simulink model "dynamics"  (R2017b)
settings: Solver=VariableStepAuto  StartTime=0.0  StopTime=10.0  RelTol=1e-3
libraries: shared6dof x1
settings Model: Creator=DanAdmin  LastModifiedBy=DanAdmin

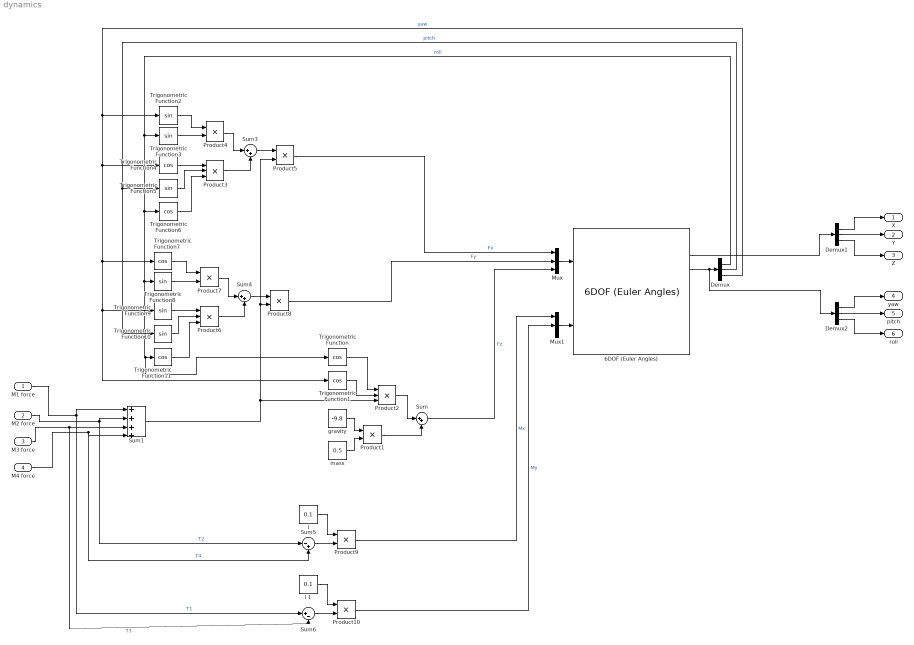
== system dynamics ==
  M1 force : Inport
  M2 force : Inport  Port=2
  M3 force : Inport  Port=3
  M4 force : Inport  Port=4
  6DOF (Euler Angles) : shared6dof/6DOF (Euler Angles)  units=Metric (MKS)  mtype=Fixed  rep=Euler Angles  xme_0=[0 0 0]  Vm_0=[0 0 0]  eul_0=[0 0 0]  pm_0=[0 0 0]  mass_0=1.0  mass_e=0.5  mass_f=2.0  inertia=eye(3)  inertia_e=eye(3)  inertia_f=2*eye(3)  k_quat=1.0  vre_flag=on  abi_flag=off
      settings: SourceProductBaseCode=AE
  Demux : Demux  Outputs=3
  Demux1 : Demux  Outputs=3
  Demux2 : Demux  Outputs=3
  Mux : Mux  Inputs=3
  Mux1 : Mux  Inputs=3
  Product{1,4..5,7..10} (7 alike) : Product
  Product2 : Product  Inputs=3
  Product3 : Product  Inputs=3
  Product6 : Product  Inputs=3
  Sum : Sum  Inputs=|++
  Sum1 : Sum  Inputs=|++++
  Sum3 : Sum  Inputs=|++
  Sum4 : Sum  Inputs=|++
  Sum5 : Sum  Inputs=|-+
  Sum6 : Sum  Inputs=|+-
  Trigonometric Function{,1,4,6..7,11} (6 alike) : Trigonometry  Operator=cos
  Trigonometric Function{2..3,5,8..10} (6 alike) : Trigonometry
  gravity : Constant  Value=-9.8
  "l " : Constant  Value=0.1
  l 1 : Constant  Value=0.1
  mass : Constant  Value=0.5
  X : Outport
  Y : Outport  Port=2
  Z : Outport  Port=3
  yaw : Outport  Port=4
  pitch : Outport  Port=5
  roll : Outport  Port=6
  wires:
  Mux/1 -> 6DOF (Euler Angles)/1
  Sum/1 -> Mux/3  "Fz"
  mass/1 -> Product1/2
  gravity/1 -> Product1/1
  Trigonometric Function/1 -> Product2/1
  Trigonometric Function1/1 -> Product2/2
  Product2/1 -> Sum/1
  6DOF (Euler Angles)/2 -> Demux1/1
  M1 force/1 -> Sum6/1, Sum1/1  "T1"
  M2 force/1 -> Sum5/1, Sum1/2  "T2"
  M4 force/1 -> Sum5/2, Sum1/4  "T4"
  Product1/1 -> Sum/2
  Product3/1 -> Sum3/2
  Product5/1 -> Mux/1  "Fx"
  Demux/1 -> Trigonometric Function/1, Trigonometric Function11/1, Trigonometric Function8/1, Trigonometric Function6/1, Trigonometric Function3/1  "roll"
  Trigonometric Function2/1 -> Product4/1
  Trigonometric Function3/1 -> Product4/2
  Product4/1 -> Sum3/1
  Trigonometric Function4/1 -> Product3/1
  Trigonometric Function5/1 -> Product3/2
  Trigonometric Function6/1 -> Product3/3
  Demux/2 -> Trigonometric Function10/1, Trigonometric Function5/1  "pitch"
  Sum3/1 -> Product5/1
  Product7/1 -> Sum4/1
  Product8/1 -> Mux/2  "Fy"
  Product6/1 -> Sum4/2
  Trigonometric Function10/1 -> Product6/2
  Sum1/1 -> Product8/2, Product5/2, Product2/3
  Trigonometric Function7/1 -> Product7/1
  Sum4/1 -> Product8/1
  Trigonometric Function8/1 -> Product7/2
  Trigonometric Function9/1 -> Product6/1
  Demux/3 -> Trigonometric Function1/1, Trigonometric Function9/1, Trigonometric Function7/1, Trigonometric Function4/1, Trigonometric Function2/1  "yaw"
  Trigonometric Function11/1 -> Product6/3
  "l "/1 -> Product9/1
  Sum5/1 -> Product9/2
  Product9/1 -> Mux1/1  "Mx"
  Mux1/1 -> 6DOF (Euler Angles)/2
  M3 force/1 -> Sum6/2, Sum1/3  "T3"
  l 1/1 -> Product10/1
  Product10/1 -> Mux1/2  "My"
  Sum6/1 -> Product10/2
  Demux1/1 -> X/1
  Demux1/2 -> Y/1
  Demux1/3 -> Z/1
  6DOF (Euler Angles)/3 -> Demux2/1, Demux/1
  Demux2/3 -> roll/1
  Demux2/1 -> yaw/1
  Demux2/2 -> pitch/1
